simulink model "comp_mdl"  (R2021b)
settings: Solver=ode1  StartTime=0.0  StopTime=5  FixedStep=0.001  MaxStep=0.1  MinStep=0.001  RelTol=1e-3  EnableMultiTasking=on
values from neighbouring files (symbols this model uses):
  A = A([2:end],[2:end])    [obsint_data.m]
  B = B([2:end],:)    [obsint_data.m]
  C = C(:,:)    [obsint_data.m]
  delta = 0.001    [obsint_data.m]    (also in outmodc_data.m)
  rho = 1    [obsint_data.m]    (also in outmodc_data.m)
  S = rpp(Ai,Bi,Eopt)    [obsint_data.m]
  x0 = zeros(1,n)    [obsint_data.m]    (also in outmodc_data.m)
  xc0 = zeros(1,n-p)    [outmodc_data.m]
undefined symbols (not defined in the file or in its folder): CA, Dhat, Hhat, L, Lam, m, n, p, P
settings Model: Creator=w.schwamm  LastModifiedBy=w.schwamm
settings SolverCC: AlgebraicLoopSolver=TrustRegion
settings DataIOCC: SaveOutput=off  SaveTime=off  ReturnWorkspaceOutputs=off  StateSaveName=x  TimeSaveName=t  OutputSaveName=y
settings OptimizationCC: LifeSpan=inf
settings DebuggingCC: SFUnexpectedBacktrackingDiag=warning  SFNoUnconditionalDefaultTransitionDiag=warning  SFMachineParentedDataDiag=warning  ArithmeticOperatorsInVariantConditions=warning
settings SFSimCC: SimUseLocalCustomCode=off  CustomCodeUndefinedFunction=UseInterfaceOnly
settings RTWCC: RTWUseLocalCustomCode=off
settings CodeAppCC: StateflowObjectComments=on
settings GRTTargetCC: TargetLangStandard=C89/C90 (ANSI)
settings ConfigComp: CovMetricSettings=dw  CovSaveCumulativeToWorkspaceVar=on  CovSaveSingleToWorkspaceVar=on  CovExternalEMLEnable=off

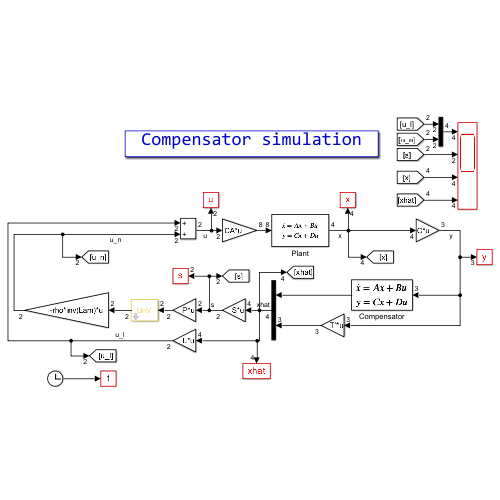
[thumbnail: Simulink's stored preview of the top-level diagram]
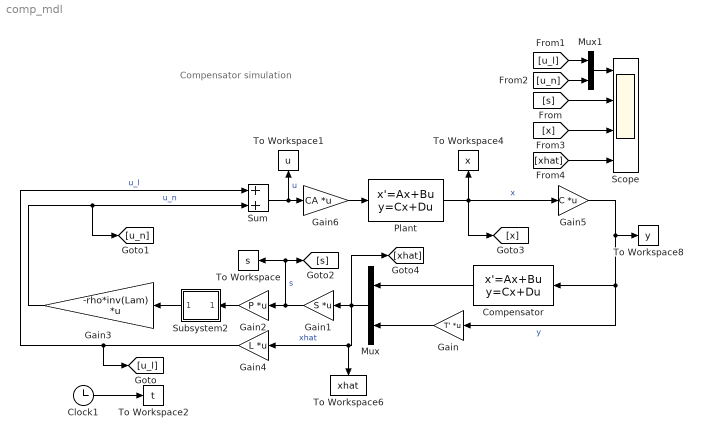
== system comp_mdl ==
  note: Compensator simulation
  Clock1 : Clock
  Compensator : StateSpace  A=Hhat  B=Dhat  C=eye(n-p)  D=zeros(n-p,p)  InitialCondition=xc0
  Gain : Gain  Gain=T'  Multiplication=Matrix(K*u)
  Gain1 : Gain  Gain=S  Multiplication=Matrix(K*u)
  Gain2 : Gain  Gain=P  Multiplication=Matrix(K*u)
  Gain3 : Gain  Gain=-rho*inv(Lam)  Multiplication=Matrix(K*u)
  Gain4 : Gain  Gain=L  Multiplication=Matrix(K*u)
  Gain5 : Gain  Gain=C  Multiplication=Matrix(K*u)
  Gain6 : Gain  Gain=CA  Multiplication=Matrix(K*u)
  Mux : Mux  Inputs=2
  Mux1 : Mux  Inputs=2
  Plant : StateSpace  A=A  B=B  C=eye(n)  D=zeros(n,m)  InitialCondition=x0
  Scope : Scope  NumInputPorts=4
  Subsystem2 : Subsystem  mask{delta=delta}
      mask prompts: delta "Unit vector delta:"
      mask Display: disp('UnV')
  Sum : Sum  InputSameDT=on  SaturateOnIntegerOverflow=on  OutDataTypeStr=Inherit: Same as first input
  To Workspace : ToWorkspace  VariableName=s  SaveFormat=Timeseries  SampleTime=-1
      settings: MaxDataPoints=1000000
  To Workspace1 : ToWorkspace  VariableName=u  SaveFormat=Timeseries  SampleTime=-1
      settings: MaxDataPoints=1000000
  To Workspace2 : ToWorkspace  VariableName=t  SaveFormat=Timeseries  SampleTime=-1
      settings: MaxDataPoints=1000000
  To Workspace4 : ToWorkspace  VariableName=x  SaveFormat=Timeseries  SampleTime=-1
      settings: MaxDataPoints=1000000
  To Workspace6 : ToWorkspace  VariableName=xhat  SaveFormat=Timeseries  SampleTime=-1
      settings: MaxDataPoints=1000000
  To Workspace8 : ToWorkspace  VariableName=y  SaveFormat=Timeseries  SampleTime=-1
      settings: MaxDataPoints=1000000
  wires:
  Plant/1 -> Gain5/1, To Workspace4/1, [x]  "x"
  Clock1/1 -> To Workspace2/1
  Gain5/1 -> Compensator/1, Gain/1, To Workspace8/1  "y"
  Subsystem2/1(Out1) -> Gain3/1
  Mux/1 -> [xhat], Gain4/1, To Workspace6/1, Gain1/1  "xhat"
  Gain/1 -> Mux/2
  Compensator/1 -> Mux/1
  Gain1/1 -> Gain2/1, To Workspace/1, [s]  "s"
  Gain2/1 -> Subsystem2/1(In1)
  Gain4/1 -> [u_l], Sum/1  "u_l"
  Gain3/1 -> [u_n], Sum/2  "u_n"
  Sum/1 -> Gain6/1, To Workspace1/1  "u"
  Mux1/1 -> Scope/1
  [s] -> Scope/2
  [u_l] -> Mux1/1
  [u_n] -> Mux1/2
  [x] -> Scope/3
  [xhat] -> Scope/4
  Gain6/1 -> Plant/1

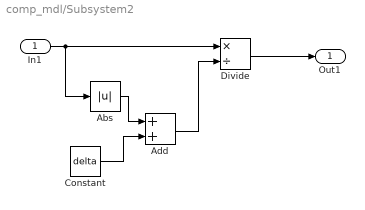
== system comp_mdl/Subsystem2 ==
  In1 : Inport
  Abs : Abs
  Add : Sum
  Constant : Constant  Value=delta  SampleTime=-1
  Divide : Product  Inputs=*/
  Out1 : Outport
  wires:
  Constant/1 -> Add/2
  Add/1 -> Divide/2
  Abs/1 -> Add/1
  Divide/1 -> Out1/1
  In1/1 -> Divide/1, Abs/1
